simulink model "Test2Part4b"  (R2024a)
settings: Solver=FixedStepAuto  StartTime=0.0  StopTime=4000  FixedStep=1  RelTol=1e-3
libraries: matrix_library x2
settings Model: Creator=katutu  LastModifiedBy=katutu

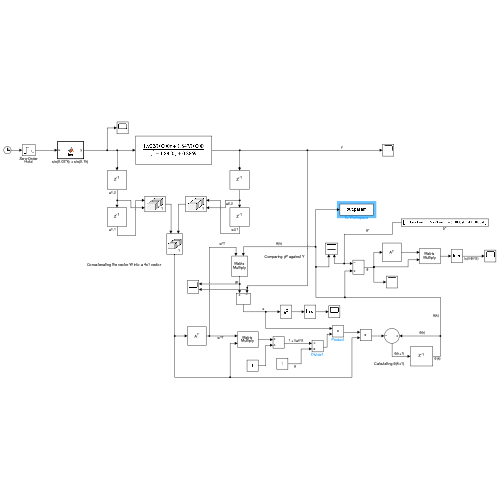
[thumbnail: Simulink's stored preview of the top-level diagram]
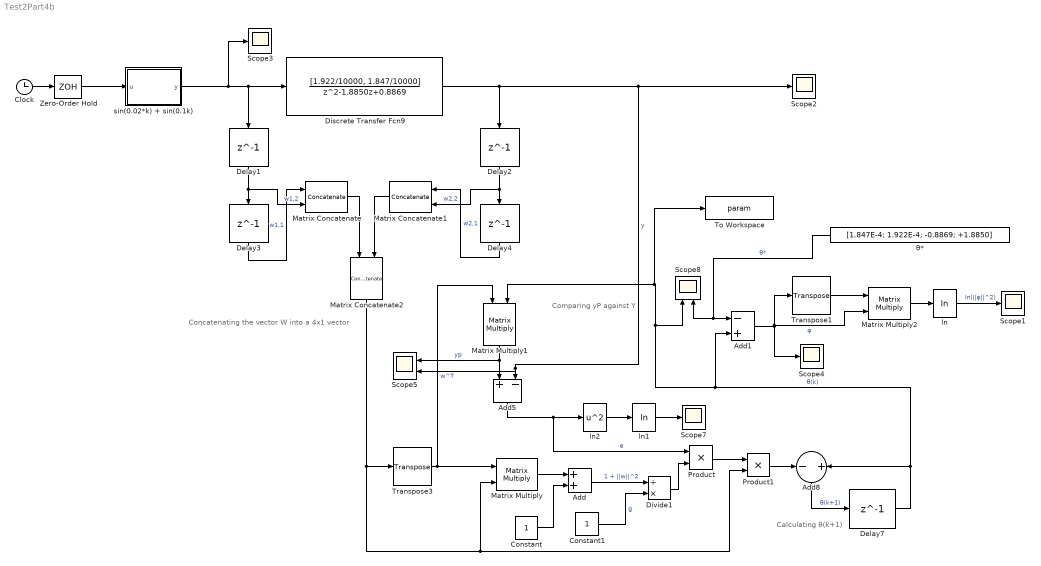
== system Test2Part4b ==
  note: Comparing yP against Y
  note: Calculating θ(k+1)
  note: Concatenating the vector W into a 4x1 vector
  Add : Sum
  Add1 : Sum  Inputs=-+
  Add5 : Sum  Inputs=+-
  Add8 : Sum  Inputs=-+
  Clock : Clock
  Constant : Constant
  Constant1 : Constant
  Delay{1..4} (4 alike) : Delay  DelayLength=1  InitialCondition=0
  Delay7 : Delay  DelayLength=1  InitialCondition=[0; 0; 0; 0]
  Discrete Transfer Fcn9 : DiscreteTransferFcn  Numerator=[1.922/10000, 1.847/10000]  Denominator=[1 -1.8850 0.8869]
  Divide1 : Product  Inputs=/*
  Matrix Concatenate : Concatenate  Mode=Multidimensional array
  Matrix Concatenate1 : Concatenate  Mode=Multidimensional array
  Matrix Concatenate2 : Concatenate  Mode=Multidimensional array
  Matrix Multiply : Product  Multiplication=Matrix(*)
  Matrix Multiply1 : Product  Multiplication=Matrix(*)
  Matrix Multiply2 : Product  Multiplication=Matrix(*)
  Product : Product
  Product1 : Product
  Scope{1..4,7} (5 alike) : Scope
  Scope5 : Scope  NumInputPorts=2
  Scope8 : Scope  NumInputPorts=2
  To Workspace : ToWorkspace  VariableName=param  SampleTime=-1
      settings: MaxDataPoints=1
  Transpose1 : matrix_library/Transpose
  Transpose3 : matrix_library/Transpose
  Zero-Order Hold : ZeroOrderHold  SampleTime=-1
  ln : Math  Operator=log
  ln1 : Math  Operator=log
  ln2 : Math  Operator=square
  sin(0.02*k) + sin(0.1k) : MATLAB Function  TreatAsAtomicUnit=on
  θ* : Constant  Value=[1.847E-4; 1.922E-4; -0.8869; +1.8850]
  wires:
  ln2/1 -> ln1/1
  Add8/1 -> Delay7/1  "θ(k+1)"
  Add5/1 -> Product/1, ln2/1  "e"
  Delay1/1 -> Matrix Concatenate/2, Delay3/1  "w1,2"
  Delay3/1 -> Matrix Concatenate/1  "w1,1"
  Matrix Multiply1/1 -> Add5/1, Scope5/1  "yp"
  Transpose3/1 -> Matrix Multiply/1, Matrix Multiply1/1  "w^T"
  sin(0.02*k) + sin(0.1k)/1(y) -> Scope3/1, Delay1/1, Discrete Transfer Fcn9/1
  Matrix Concatenate2/1 -> Matrix Multiply/2, Product1/2, Transpose3/1
  Delay4/1 -> Matrix Concatenate1/1  "w2,1"
  Delay2/1 -> Matrix Concatenate1/2, Delay4/1  "w2,2"
  Product1/1 -> Add8/1
  Clock/1 -> Zero-Order Hold/1
  ln/1 -> Scope1/1  "ln(||φ||^2)"
  Zero-Order Hold/1 -> sin(0.02*k) + sin(0.1k)/1(u)
  Add1/1 -> Transpose1/1, Matrix Multiply2/2, Scope4/1  "φ"
  θ*/1 -> Add1/1, Scope8/2  "θ*"
  Discrete Transfer Fcn9/1 -> Delay2/1, Scope2/1, Scope5/2, Add5/2  "y"
  Matrix Concatenate1/1 -> Matrix Concatenate2/2
  Matrix Concatenate/1 -> Matrix Concatenate2/1
  ln1/1 -> Scope7/1
  Delay7/1 -> To Workspace/1, Matrix Multiply1/2, Scope8/1, Add1/2, Add8/2  "θ(k)"
  Matrix Multiply/1 -> Add/1
  Constant/1 -> Add/2
  Add/1 -> Divide1/1  "1 + ||w||^2"
  Constant1/1 -> Divide1/2  "g"
  Divide1/1 -> Product/2
  Product/1 -> Product1/1
  Transpose1/1 -> Matrix Multiply2/1
  Matrix Multiply2/1 -> ln/1

== matlab function Test2Part4b/sin(0.02*k) + sin(0.1k) ==
  data: u input; y output
function y = fcn(u)

y = sin(0.02*u) + sin(0.1*u);
